simulink model "Antriebsstrangmodell_V1_4_n5"  (R2019a)
settings: Solver=FixedStepAuto  StartTime=0.0  StopTime=t_Simulation  FixedStep=dt  RelTol=1e-3
values from neighbouring files (symbols this model uses):
  A_Stirn = 2    [SIMULA~1.M]    (also in SIMULA~2.M)
  alpha_Luft = -4e-3    (= -0.004)    [SIMULA~1.M]    (also in SIMULA~2.M)
  alpha_Rotor = alpha_Al    (= 0.004)    [SIMULA~1.M]    (also in SIMULA~2.M)
  alpha_Stator = alpha_Al    (= 0.004)    [SIMULA~1.M]    (also in SIMULA~2.M)
  alpha_Ummag = -0.75e-3    (= -0.00075)    [SIMULA~1.M]    (also in SIMULA~2.M)
  c_W = 0.37    [SIMULA~1.M]    (also in SIMULA~2.M)
  COG_x = 1.4267    [SIMULA~1.M]    (also in SIMULA~2.M)
  COG_z = 0.4572    [SIMULA~1.M]    (also in SIMULA~2.M)
  cp_Luft = 1008.8    [SIMULA~1.M]    (also in SIMULA~2.M)
  e_Fahrzeug = 1.0478    [SIMULA~1.M]    (also in SIMULA~2.M)
  eta_EMaschine_Break_M_EMaschine = flipud(KennfeldMaschine.M(:,1))'    [SIMULA~1.M]    (also in SIMULA~2.M)
  eta_EMaschine_Break_M_EMaschine_reku = -KennfeldMaschine.M(:,1)'    [SIMULA~1.M]    (also in SIMULA~2.M)
  eta_EMaschine_Break_n_EMaschine = KennfeldMaschine.n(end-1,:)    [SIMULA~1.M]    (also in SIMULA~2.M)
  eta_EMaschine_Break_n_EMaschine_reku = KennfeldMaschine.n(end-1,:)    [SIMULA~1.M]    (also in SIMULA~2.M)
  eta_EMaschine_Faktor_Volllast = 0.98    [SIMULA~1.M]    (also in SIMULA~2.M)
  eta_EMaschine_Table = flip(KennfeldMaschine.etages,1)    [SIMULA~1.M]    (also in SIMULA~2.M)
  eta_EMaschine_Table_reku = KennfeldMaschine.etages    [SIMULA~1.M]    (also in SIMULA~2.M)
  eta_Getriebe = 0.96    [SIMULA~1.M]    (also in SIMULA~2.M)
  eta_IA = 0.5    [SIMULA~1.M]    (also in SIMULA~2.M)
  h_WC_pumpoff = Nu_WC*lam_WC/dh_WC    [SIMULA~1.M]    (also in SIMULA~2.M)
  h_WC_pumpon = Nu_WC*lam_WC/dh_WC    [SIMULA~1.M]    (also in SIMULA~2.M)
  i_Getriebe = 5.697    [SIMULA~1.M]    (also in SIMULA~2.M)
  krb_Korrektur = 0.53/10    (= 0.053)    [SIMULA~1.M]    (also in SIMULA~2.M)
  lam_Luft = 0.028592    [SIMULA~1.M]    (also in SIMULA~2.M)
  M_EMaschine_max = zeros(2,numel(eta_EMaschine_Break_n_EMaschine))    [SIMULA~1.M]    (also in SIMULA~2.M)
  m_Fahrzeug = 825    [SIMULA~1.M]    (also in SIMULA~2.M)
  m_Zuladung = 80    [SIMULA~1.M]    (also in SIMULA~2.M)
  nue_Luft = 19.230034390524e-6    (= 1.92300343905e-05)    [SIMULA~1.M]    (also in SIMULA~2.M)
  pump_start_limit = 273.15 + 33    (= 306.15)    [SIMULA~1.M]    (also in SIMULA~2.M)
  r_dynamisch = 0.2774    [SIMULA~1.M]    (also in SIMULA~2.M)
  rho_Luft = 1.2    [SIMULA~1.M]    (also in SIMULA~2.M)
  rho_Luft_EM = 1.0468    [SIMULA~1.M]    (also in SIMULA~2.M)
  share_EMaschine_Ummagnet_reku_Table = ser.gen.share_Ummagnetisierungsverluste    [SIMULA~1.M]    (also in SIMULA~2.M)
  share_EMaschine_Ummagnet_Table = ser.mot.share_Ummagnetisierungsverluste    [SIMULA~1.M]    (also in SIMULA~2.M)
  share_EMaschine_Wicklung_reku_Table = ser.gen.share_Wicklungsverluste    [SIMULA~1.M]    (also in SIMULA~2.M)
  share_EMaschine_Wicklung_Table = ser.mot.share_Wicklungsverluste    [SIMULA~1.M]    (also in SIMULA~2.M)
  share_EMaschine_WirkMech_reku_Table = ser.gen.share_WirkmechVerluste    [SIMULA~1.M]    (also in SIMULA~2.M)
  share_EMaschine_WirkMech_Table = ser.mot.share_WirkmechVerluste    [SIMULA~1.M]    (also in SIMULA~2.M)
  share_EMaschine_WirkZus_reku_Table = ser.gen.share_WirkZusVerl    [SIMULA~1.M]    (also in SIMULA~2.M)
  share_EMaschine_WirkZus_Table = ser.mot.share_WirkZusVerl    [SIMULA~1.M]    (also in SIMULA~2.M)
  T_Entwurf_Rotor = 273.15+20    (= 293.15)    [SIMULA~1.M]    (also in SIMULA~2.M)
  T_Entwurf_Stator = 273.15+20    (= 293.15)    [SIMULA~1.M]    (also in SIMULA~2.M)
  t_Simulation = v_Fahrzeug.Time(end)+1    [SIMULA~1.M]    (also in SIMULA~2.M = v_Fahrzeug.Time(end))
  T_Start_EMaschine = 273.15 + 23    (= 296.15)    [SIMULA~1.M]    (also in SIMULA~2.M)
  v_max = 110    [SIMULA~1.M]    (also in SIMULA~2.M)
  WB = 2.96    [SIMULA~1.M]    (also in SIMULA~2.M)
undefined symbols (not defined in the file or in its folder): A_AGP, A_IA, Anteil_Rotor_Ringe, Anteil_Stator, chi_Lager, D_2a, D_2r, delta, f_R, m_RTO, m_RYO, m_SSL_L, m_STO, m_SYO, m_WH_L, n_dis
libraries: fl_lib x440, nesl_utility x106, SimscapeCustomBlocks_lib x45, simulink x3
(part 1 of 5)
settings Model: Creator=Ludwig Stolle  LastModifiedBy=Ludwig Stolle
settings DataIOCC: SaveOutput=off  SignalLogging=off  DSMLogging=off  SaveTime=off  ReturnWorkspaceOutputs=off
settings DebuggingCC: UnconnectedInputMsg=none  UnconnectedOutputMsg=none

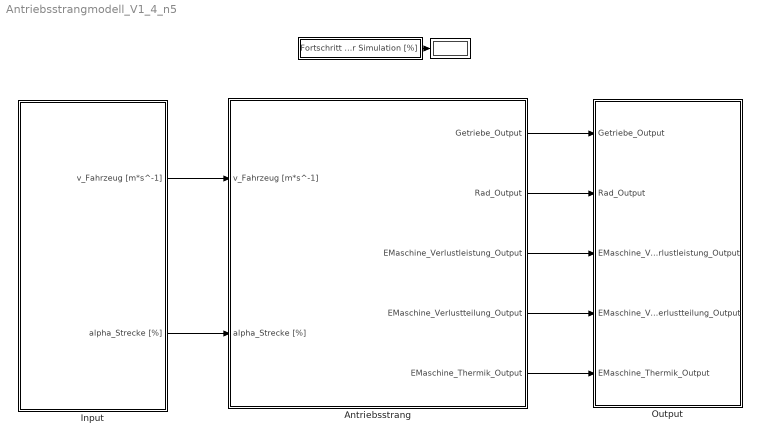
== system Antriebsstrangmodell_V1_4_n5 ==
  "\t\t     " : Subsystem
  " " : Display
      settings: Format=bank
  Antriebsstrang : Subsystem
  Input : Subsystem
  Output : Subsystem
  wires:
  Input/1(v_Fahrzeug [m*s^-1]) -> Antriebsstrang/1(v_Fahrzeug [m*s^-1])
  Input/2(alpha_Strecke [%]) -> Antriebsstrang/2(alpha_Strecke [%])
  Antriebsstrang/1(Getriebe_Output) -> Output/1(Getriebe_Output)
  Antriebsstrang/2(Rad_Output) -> Output/2(Rad_Output)
  "\t\t     "/1(Fortschritt der Simulation [%]) -> " "/1
  Antriebsstrang/3(EMaschine_Verlustleistung_Output) -> Output/3(EMaschine_Verlustleistung_Output)
  Antriebsstrang/4(EMaschine_Verlustteilung_Output) -> Output/4(EMaschine_Verlustteilung_Output)
  Antriebsstrang/5(EMaschine_Thermik_Output) -> Output/5(EMaschine_Thermik_Output)

== system Antriebsstrangmodell_V1_4_n5/		      ==
  note: Fortschritt der Simulation = 100 * simulierte Zeit / t_Simulation
      |
      | mit Fortschritt der Simulation in %
  Clock : Clock
  Constant : Constant  Value=t_Simulation  VectorParams1D=off
  Divide : Product  Inputs=*/
  Umrechnung in % : Gain  Gain=100
  Fortschritt der Simulation [%] : Outport
  wires:
  Constant/1 -> Divide/2
  Clock/1 -> Divide/1
  Divide/1 -> Umrechnung in %/1
  Umrechnung in %/1 -> Fortschritt der Simulation [%]/1

== system Antriebsstrangmodell_V1_4_n5/Antriebsstrang ==
  v_Fahrzeug [m*s^-1] : Inport
  alpha_Strecke [%] : Inport  Port=2
  E-Maschine Thermik : Subsystem
  E-Maschine Verlustleistung : Subsystem
  E-Maschine Verlustteilung : Subsystem
  Getriebe : Subsystem
  Rad : Subsystem
  Getriebe_Output : Outport
  Rad_Output : Outport  Port=2
  EMaschine_Verlustleistung_Output : Outport  Port=3
  EMaschine_Verlustteilung_Output : Outport  Port=4
  EMaschine_Thermik_Output : Outport  Port=5
  wires:
  alpha_Strecke [%]/1 -> Rad/2(alpha_Strecke [%])
  v_Fahrzeug [m*s^-1]/1 -> Rad/1(v_Fahrzeug [m*s^-1])
  Rad/1(Rad_Output) -> Rad_Output/1, Getriebe/1(Rad_Output)
  Getriebe/1(Getriebe_Output) -> Getriebe_Output/1, E-Maschine Verlustleistung/1(Getriebe_Output), E-Maschine Verlustteilung/2(Getriebe_Output), E-Maschine Thermik/2(Getriebe_Output)
  E-Maschine Verlustleistung/1(EMaschine_Verlustleistung_Output) -> EMaschine_Verlustleistung_Output/1, E-Maschine Verlustteilung/1(EMaschine_Verlustleistung_Output)
  E-Maschine Verlustteilung/1(EMaschine_Verlustteilung_Output) -> EMaschine_Verlustteilung_Output/1, E-Maschine Thermik/1(EMaschine_Verlustlteilung_Output)
  E-Maschine Thermik/1(EMaschine_Thermik_Output) -> EMaschine_Thermik_Output/1
  E-Maschine Verlustleistung/2(Regelabweichung [Nm]) -> Rad/3(Regelabweichung [Nm])

== system Antriebsstrangmodell_V1_4_n5/Input ==
  note: Umrechnung km/h in m/s
  note: Nur positive Geschwindigkeit
  From Workspace : FromWorkspace  VariableName=v_Fahrzeug  SampleTime=0  OutputAfterFinalValue=Setting to zero
  From Workspace1 : FromWorkspace  VariableName=alpha_Strecke  SampleTime=0  OutputAfterFinalValue=Setting to zero
  Gain : Gain  Gain=1/3.6
  Saturation : Saturate  UpperLimit=v_max  LowerLimit=0
  v_Fahrzeug [m*s^-1] : Outport
  alpha_Strecke [%] : Outport  Port=2
  wires:
  Saturation/1 -> Gain/1
  From Workspace/1 -> Saturation/1
  Gain/1 -> v_Fahrzeug [m*s^-1]/1
  From Workspace1/1 -> alpha_Strecke [%]/1

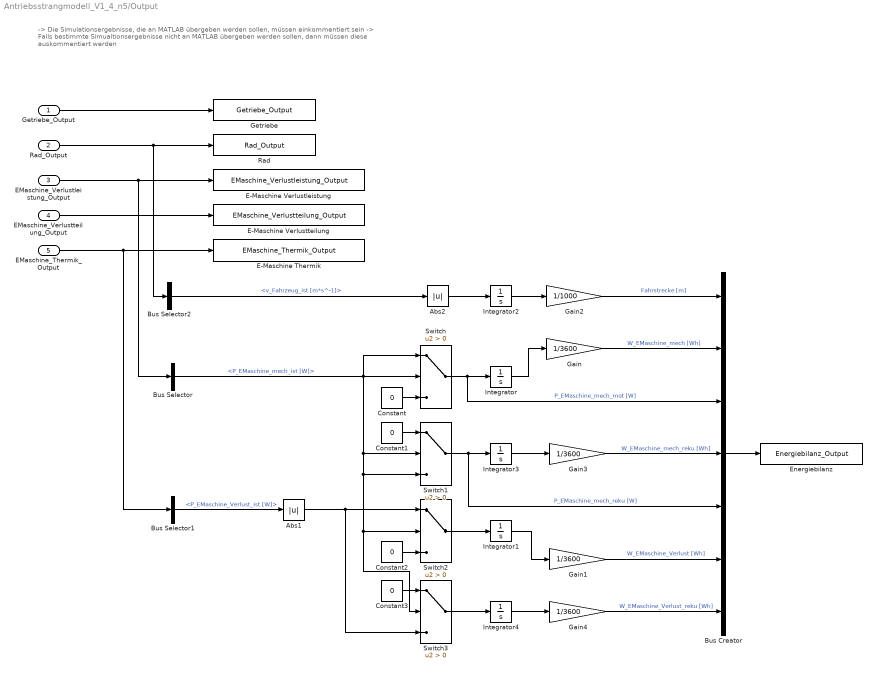
== system Antriebsstrangmodell_V1_4_n5/Output ==
  note: -> Die Simulationsergebnisse, die an MATLAB übergeben werden sollen, müssen einkommentiert sein
      | -> Falls bestimmte Simualtionsergebnisse nicht an MATLAB übergeben werden sollen, dann müssen diese auskommentiert werden
  Getriebe_Output : Inport
  Rad_Output : Inport  Port=2
  EMaschine_Verlustleistung_Output : Inport  Port=3
  EMaschine_Verlustteilung_Output : Inport  Port=4
  EMaschine_Thermik_Output : Inport  Port=5
  Abs1 : Abs
  Abs2 : Abs
  Bus Creator : BusCreator  Inputs=7
  Bus Selector : BusSelector  OutputSignals=P_EMaschine_mech_ist [W]
  Bus Selector1 : BusSelector  OutputSignals=P_EMaschine_Verlust_ist [W]
  Bus Selector2 : BusSelector  OutputSignals=v_Fahrzeug_ist [m*s^-1]
  Constant{,1..3} (4 alike) : Constant  Value=0
  E-Maschine Thermik : ToWorkspace  VariableName=EMaschine_Thermik_Output  SaveFormat=Timeseries  SampleTime=-1
      settings: Decimation=Decimation_Output
  E-Maschine Verlustleistung : ToWorkspace  VariableName=EMaschine_Verlustleistung_Output  SaveFormat=Timeseries  SampleTime=-1
      settings: Decimation=Decimation_Output
  E-Maschine Verlustteilung : ToWorkspace  VariableName=EMaschine_Verlustteilung_Output  SaveFormat=Timeseries  SampleTime=-1
      settings: Decimation=Decimation_Output
  Energiebilanz : ToWorkspace  VariableName=Energiebilanz_Output  SaveFormat=Timeseries  SampleTime=-1
      settings: Decimation=Decimation_Output
  Gain{,1,3..4} (4 alike) : Gain  Gain=1/3600
  Gain2 : Gain  Gain=1/1000
  Getriebe : ToWorkspace  VariableName=Getriebe_Output  SaveFormat=Timeseries  SampleTime=-1
      settings: Decimation=Decimation_Output
  Integrator{,1..4} (5 alike) : Integrator
  Rad : ToWorkspace  VariableName=Rad_Output  SaveFormat=Timeseries  SampleTime=-1
      settings: Decimation=Decimation_Output
  Switch{,1..3} (4 alike) : Switch  Criteria=u2 > Threshold
  wires:
  Getriebe_Output/1 -> Getriebe/1
  Rad_Output/1 -> Rad/1, Bus Selector2/1
  EMaschine_Verlustleistung_Output/1 -> E-Maschine Verlustleistung/1, Bus Selector/1
  EMaschine_Verlustteilung_Output/1 -> E-Maschine Verlustteilung/1
  EMaschine_Thermik_Output/1 -> E-Maschine Thermik/1, Bus Selector1/1
  Bus Selector1/1 -> Abs1/1  "<P_EMaschine_Verlust_ist [W]>"
  Integrator/1 -> Gain/1
  Integrator1/1 -> Gain1/1
  Bus Selector/1 -> Switch/2, Switch3/2, Switch2/2, Switch1/3, Switch1/2, Switch/1  "<P_EMaschine_mech_ist [W]>"
  Bus Creator/1 -> Energiebilanz/1
  Gain/1 -> Bus Creator/2  "W_EMaschine_mech [Wh]"
  Gain2/1 -> Bus Creator/1  "Fahrstrecke [m]"
  Bus Selector2/1 -> Abs2/1  "<v_Fahrzeug_ist [m*s^-1]>"
  Integrator2/1 -> Gain2/1
  Abs2/1 -> Integrator2/1
  Switch/1 -> Bus Creator/3, Integrator/1  "P_EMaschine_mech_mot [W]"
  Constant/1 -> Switch/3
  Constant1/1 -> Switch1/1
  Switch1/1 -> Bus Creator/5, Integrator3/1  "P_EMaschine_mech_reku [W]"
  Integrator3/1 -> Gain3/1
  Gain3/1 -> Bus Creator/4  "W_EMaschine_mech_reku [Wh]"
  Abs1/1 -> Switch3/3, Switch2/1
  Switch2/1 -> Integrator1/1
  Constant2/1 -> Switch2/3
  Gain1/1 -> Bus Creator/6  "W_EMaschine_Verlust [Wh]"
  Constant3/1 -> Switch3/1
  Integrator4/1 -> Gain4/1
  Switch3/1 -> Integrator4/1
  Gain4/1 -> Bus Creator/7  "W_EMaschine_Verlust_reku [Wh]"

== system Antriebsstrangmodell_V1_4_n5/Antriebsstrang/E-Maschine Thermik ==
  EMaschine_Verlustlteilung_Output : Inport
  Getriebe_Output : Inport  Port=2
  Aufteilung mechanischer Verluste auf Lager & Lüftung : Subsystem
  Bus Creator : BusCreator  Inputs=15
  Bus Selector1 : BusSelector  OutputSignals=P_EMaschine_Verlust_Wicklung [W],P_EMaschine_Verlust_Ummagnet [W],P_EMaschine_Verlust_WirkZus [W],P_EMaschine_Verlust_WirkMech [W]
  Bus Selector2 : BusSelector  OutputSignals=n_EMaschine [min^-1]
  Thermisches Netzwerk : Subsystem
  Wärmeübergangskoeffizienten Konvektion Luftspalt und Endcap-Luft : Subsystem
  EMaschine_Thermik_Output : Outport
  wires:
  EMaschine_Verlustlteilung_Output/1 -> Bus Selector1/1
  Getriebe_Output/1 -> Bus Selector2/1
  Bus Creator/1 -> EMaschine_Thermik_Output/1
  Bus Selector2/1 -> Wärmeübergangskoeffizienten Konvektion Luftspalt und Endcap-Luft/1(<n_EMaschine [min^-1]>), Aufteilung mechanischer Verluste auf Lager & Lüftung/2(n_EMaschine [min^-1])  "<n_EMaschine [min^-1]>"
  Bus Selector1/2 -> Thermisches Netzwerk/2(P_EMaschine_Verlust_Ummagnet [W])  "<P_EMaschine_Verlust_Ummagnet [W]>"
  Bus Selector1/3 -> Thermisches Netzwerk/3(P_EMaschine_Verlust_WirkZus [W])  "<P_EMaschine_Verlust_WirkZus [W]>"
  Bus Selector1/1 -> Thermisches Netzwerk/1(P_EMaschine_Verlust_Wicklung [W])  "<P_EMaschine_Verlust_Wicklung [W]>"
  Wärmeübergangskoeffizienten Konvektion Luftspalt und Endcap-Luft/1(HTC_Luftspalt [W*m^-2*K^-1]) -> Thermisches Netzwerk/6(HTC_Luftspalt [W*m^-2*K^-1])
  Aufteilung mechanischer Verluste auf Lager & Lüftung/1(P_EMaschine_Verlust_Lueftung [W]) -> Thermisches Netzwerk/4(P_EMaschine_Verlust_Lueftung [W])
  Bus Selector1/4 -> Aufteilung mechanischer Verluste auf Lager & Lüftung/1(P_EMaschine_Verlust_WirkMech [W])  "<P_EMaschine_Verlust_WirkMech [W]>"
  Aufteilung mechanischer Verluste auf Lager & Lüftung/2(P_EMaschine_Verlust_Lager [W]) -> Thermisches Netzwerk/5(P_EMaschine_Verlust_Lager [W])
  Thermisches Netzwerk/1(T_EMaschine_WH [K]) -> Bus Creator/1
  Thermisches Netzwerk/2(T_EMaschine_Kuehlmittel [K]) -> Bus Creator/2
  Thermisches Netzwerk/3(T_EMaschine_SSL [K]) -> Bus Creator/3
  Thermisches Netzwerk/4(T_EMaschine_ER [K]) -> Bus Creator/4
  Thermisches Netzwerk/5(P_EMaschine_Verlust_ist [W]) -> Bus Creator/5
  Thermisches Netzwerk/6(T_EMaschine_STO [K]) -> Bus Creator/6
  Thermisches Netzwerk/7(T_EMaschine_AGP [K]) -> Bus Creator/7
  Thermisches Netzwerk/8(T_EMaschine_SYO [K]) -> Bus Creator/8
  Thermisches Netzwerk/9(T_EMaschine_RSL [K]) -> Bus Creator/9
  Thermisches Netzwerk/11(T_EMaschine_RYO [K]) -> Bus Creator/11
  Thermisches Netzwerk/10(T_EMaschine_RTO [K]) -> Bus Creator/10
  Wärmeübergangskoeffizienten Konvektion Luftspalt und Endcap-Luft/2(HTC_fconv_Luftspalt [W*m^-2*K^-1]) -> Thermisches Netzwerk/7(HTC_fconv_Luftspalt [W*m^-2*K^-1])
  Wärmeübergangskoeffizienten Konvektion Luftspalt und Endcap-Luft/4(HTC_fconv_Innenluft [W*m^-2*K^-1]) -> Thermisches Netzwerk/9(HTC_fconv_Innenluft [W*m^-2*K^-1])
  Thermisches Netzwerk/12(T_EMaschine_IA [K]) -> Bus Creator/12
  Thermisches Netzwerk/13(T_EMaschine_SH [K]) -> Bus Creator/13
  Thermisches Netzwerk/14(T_EMaschine_HO [K]) -> Bus Creator/14
  Thermisches Netzwerk/15(T_EMaschine_EC [K]) -> Bus Creator/15
  Wärmeübergangskoeffizienten Konvektion Luftspalt und Endcap-Luft/3(HTC_Innenluft [W*m^-2*K^-1]) -> Thermisches Netzwerk/8(HTC_Innenluft [W*m^-2*K^-1])

== system Antriebsstrangmodell_V1_4_n5/Antriebsstrang/E-Maschine Verlustleistung ==
  Getriebe_Output : Inport
  Bus Creator : BusCreator  Inputs=6
  Bus Creator1 : BusCreator  Inputs=6
  Bus Selector : BusSelector  OutputSignals=P_EMaschine_Verlust_korr [W]
  Bus Selector1 : BusSelector  OutputSignals=M_EMaschine [Nm],n_EMaschine [min^-1]
  Compare To Zero : simulink/Logic and Bit Operations/Compare To Zero  relop=>=  OutDataTypeStr=boolean
  Scope : Scope  Commented=on  NumInputPorts=3
  Switch : Switch  Criteria=u2 ~= 0
  Wikrungsgrad und Verlustleistung - Antrieb : Subsystem
  Wikrungsgrad und Verlustleistung - Rekuperation : Subsystem
  EMaschine_Verlustleistung_Output : Outport
  Regelabweichung [Nm] : Outport  Port=2
  wires:
  Getriebe_Output/1 -> Bus Selector1/1
  Bus Selector1/1 -> Wikrungsgrad und Verlustleistung - Antrieb/1(M_EMaschine [Nm]), Compare To Zero/1, Wikrungsgrad und Verlustleistung - Rekuperation/1(M_EMaschine [Nm])  "<M_EMaschine [Nm]>"
  Bus Selector1/2 -> Wikrungsgrad und Verlustleistung - Antrieb/2(n_EMaschine [min^-1]), Wikrungsgrad und Verlustleistung - Rekuperation/2(n_EMaschine [min^-1])  "<n_EMaschine [min^-1]>"
  Wikrungsgrad und Verlustleistung - Antrieb/1(eta_EMaschine [%]) -> Bus Creator/1
  Wikrungsgrad und Verlustleistung - Antrieb/2(P_Leistungselektronik [W]) -> Bus Creator/2
  Wikrungsgrad und Verlustleistung - Antrieb/3(P_EMaschine_Verlust_korr [W]) -> Scope/2, Bus Creator/3
  Wikrungsgrad und Verlustleistung - Rekuperation/1(eta_EMaschine [%]) -> Bus Creator1/1
  Wikrungsgrad und Verlustleistung - Rekuperation/2(P_Leistungselektronik [W]) -> Bus Creator1/2
  Wikrungsgrad und Verlustleistung - Rekuperation/3(P_EMaschine_Verlust_korr [W]) -> Scope/3, Bus Creator1/3
  Bus Creator/1 -> Switch/1
  Bus Creator1/1 -> Switch/3
  Compare To Zero/1 -> Switch/2
  Switch/1 -> Bus Selector/1, EMaschine_Verlustleistung_Output/1
  Bus Selector/1 -> Scope/1  "<P_EMaschine_Verlust_korr [W]>"
  Wikrungsgrad und Verlustleistung - Antrieb/4(P_EMaschine_mech_ist [W]) -> Bus Creator/4
  Wikrungsgrad und Verlustleistung - Rekuperation/4(P_EMaschine_mech_ist [W]) -> Bus Creator1/4
  Wikrungsgrad und Verlustleistung - Antrieb/6(Regelabweichung [Nm]) -> Regelabweichung [Nm]/1, Bus Creator/6, Bus Creator1/6
  Wikrungsgrad und Verlustleistung - Antrieb/5(M_EMaschine_ist [Nm]) -> Bus Creator/5
  Wikrungsgrad und Verlustleistung - Rekuperation/5(M_EMaschine_ist [Nm]) -> Bus Creator1/5

== system Antriebsstrangmodell_V1_4_n5/Antriebsstrang/E-Maschine Verlustteilung ==
  EMaschine_Verlustleistung_Output : Inport
  Getriebe_Output : Inport  Port=2
  Bus Creator : BusCreator  Inputs=4
  Bus Creator1 : BusCreator  Inputs=4
  Bus Selector1 : BusSelector  OutputSignals=P_EMaschine_Verlust_korr [W]
  Bus Selector2 : BusSelector  OutputSignals=M_EMaschine [Nm],n_EMaschine [min^-1]
  Bus Selector3 : BusSelector  Commented=on  OutputSignals=P_Verlust_EMaschine_Wicklung [W],P_Verlust_EMaschine_WirkMech [W]
  Bus Selector4 : BusSelector  Commented=on  OutputSignals=P_Verlust_EMaschine_Wicklung [W],P_Verlust_EMaschine_WirkMech [W]
  Compare To Zero : simulink/Logic and Bit Operations/Compare To Zero  relop=>=  OutDataTypeStr=boolean
  Demux : Demux  Commented=on
  Scope : Scope  Commented=on  NumInputPorts=5
  Scope1 : Scope  Commented=on  NumInputPorts=4
  Switch : Switch  Criteria=u2 ~= 0
  Verlustteilung EMaschine - Antrieb : Subsystem
  Verlustteilung EMaschine - Rekuperation : Subsystem
  EMaschine_Verlustteilung_Output : Outport
  wires:
  EMaschine_Verlustleistung_Output/1 -> Bus Selector1/1
  Getriebe_Output/1 -> Bus Selector2/1
  Bus Selector1/1 -> Verlustteilung EMaschine - Rekuperation/1(<P_Verlust_EMaschine [W]>), Verlustteilung EMaschine - Antrieb/1(<P_Verlust_EMaschine_korr [W]>)  "<P_EMaschine_Verlust_korr [W]>"
  Bus Selector2/1 -> Verlustteilung EMaschine - Rekuperation/2(<M_EMaschine [Nm]>), Compare To Zero/1, Verlustteilung EMaschine - Antrieb/2(<M_EMaschine [Nm]>)  "<M_EMaschine [Nm]>"
  Bus Selector2/2 -> Verlustteilung EMaschine - Antrieb/3(<n_EMaschine [min^-1]>), Verlustteilung EMaschine - Rekuperation/3(<n_EMaschine [min^-1]>)  "<n_EMaschine [min^-1]>"
  Verlustteilung EMaschine - Antrieb/1(P_EMaschine_Verlust_Wicklung [W]) -> Bus Creator/1
  Verlustteilung EMaschine - Antrieb/2(P_EMaschine_Verlust_Ummagnet [W]) -> Bus Creator/2
  Verlustteilung EMaschine - Antrieb/3(P_EMaschine_Verlust_WirkZus [W]) -> Bus Creator/3
  Compare To Zero/1 -> Switch/2
  Switch/1 -> EMaschine_Verlustteilung_Output/1
  Bus Creator/1 -> Switch/1
  Verlustteilung EMaschine - Rekuperation/1(P_EMaschine_Verlust_Wicklung [W]) -> Bus Creator1/1
  Verlustteilung EMaschine - Rekuperation/2(P_EMaschine_Verlust_Ummagnet [W]) -> Bus Creator1/2
  Verlustteilung EMaschine - Rekuperation/3(P_EMaschine_Verlust_WirkZus [W]) -> Bus Creator1/3
  Bus Creator1/1 -> Switch/3
  Demux/4 -> Scope/5
  Demux/1 -> Scope/2
  Demux/2 -> Scope/3
  Demux/3 -> Scope/4
  Bus Selector3/1 -> Scope1/1  "<P_Verlust_EMaschine_Wicklung [W]>"
  Bus Selector4/1 -> Scope1/2  "<P_Verlust_EMaschine_Wicklung [W]>"
  Bus Selector3/2 -> Scope1/3  "<P_Verlust_EMaschine_WirkMech [W]>"
  Bus Selector4/2 -> Scope1/4  "<P_Verlust_EMaschine_WirkMech [W]>"
  Verlustteilung EMaschine - Rekuperation/4(P_EMaschine_Verlust_WirkMech [W]) -> Bus Creator1/4  "P_EMaschine_Verlust_WirkMech [W]"
  Verlustteilung EMaschine - Antrieb/4(P_EMaschine_Verlust_WirkMech [W]) -> Bus Creator/4  "P_EMaschine_Verlust_WirkMech [W]"

== system Antriebsstrangmodell_V1_4_n5/Antriebsstrang/Getriebe ==
  note: Schalter für S1-Betrieb umlegen!
  note: Momentenvorgabe für S1-Kennfeld Berechnung.
  Rad_Output : Inport
  Antreiben : Subsystem
  Bus Creator : BusCreator  Inputs=4
  Bus Creator1 : BusCreator  Inputs=4
  Bus Creator2 : BusCreator  Inputs=4
  Bus Selector : BusSelector  OutputSignals=n_Rad [min^-1],M_Rad [Nm],P_Rad [W]
  Bus Selector1 : BusSelector  OutputSignals=n_EMaschine [min^-1],P_EMaschine [W],P_Verlust_Getriebe [W],M_EMaschine [Nm]
  Compare To Zero : simulink/Logic and Bit Operations/Compare To Zero  relop=>=  OutDataTypeStr=boolean
  From Workspace1 : FromWorkspace  VariableName=M_EM  SampleTime=0  OutputAfterFinalValue=Setting to zero
  Manual Switch : ManualSwitch
  Rekuperieren : Subsystem
  Switch : Switch  Criteria=u2 ~= 0
  Getriebe_Output : Outport
  wires:
  Rad_Output/1 -> Bus Selector/1
  Bus Selector/1 -> Rekuperieren/1(n_Rad [min^-1]), Antreiben/1(n_Rad [min^-1])  "<n_Rad [min^-1]>"
  Bus Selector/2 -> Compare To Zero/1, Rekuperieren/2(M_Rad [Nm]), Antreiben/2(M_Rad [Nm])  "<M_Rad [Nm]>"
  Bus Selector/3 -> Rekuperieren/3(P_Rad [W]), Antreiben/3(P_Rad [W])  "<P_Rad [W]>"
  Antreiben/1(n_EMaschine [min^-1]) -> Bus Creator/1
  Antreiben/2(M_EMaschine [Nm]) -> Bus Creator/2
  Antreiben/3(P_EMaschine [W]) -> Bus Creator/3
  Antreiben/4(P_Verlust_Getriebe [W]) -> Bus Creator/4
  Rekuperieren/3(P_EMaschine [W]) -> Bus Creator1/3
  Rekuperieren/1(n_EMaschine [min^-1]) -> Bus Creator1/1
  Rekuperieren/4(P_Verlust_Getriebe [W]) -> Bus Creator1/4
  Rekuperieren/2(M_EMaschine [Nm]) -> Bus Creator1/2
  Compare To Zero/1 -> Switch/2
  Bus Creator/1 -> Switch/1
  Bus Creator1/1 -> Switch/3
  Switch/1 -> Bus Selector1/1
  Bus Selector1/4 -> Manual Switch/1  "<M_EMaschine [Nm]>"
  Manual Switch/1 -> Bus Creator2/4  "M_EMaschine [Nm]"
  Bus Selector1/1 -> Bus Creator2/1  "<n_EMaschine [min^-1]>"
  Bus Selector1/2 -> Bus Creator2/2  "<P_EMaschine [W]>"
  Bus Selector1/3 -> Bus Creator2/3  "<P_Verlust_Getriebe [W]>"
  Bus Creator2/1 -> Getriebe_Output/1
  From Workspace1/1 -> Manual Switch/2

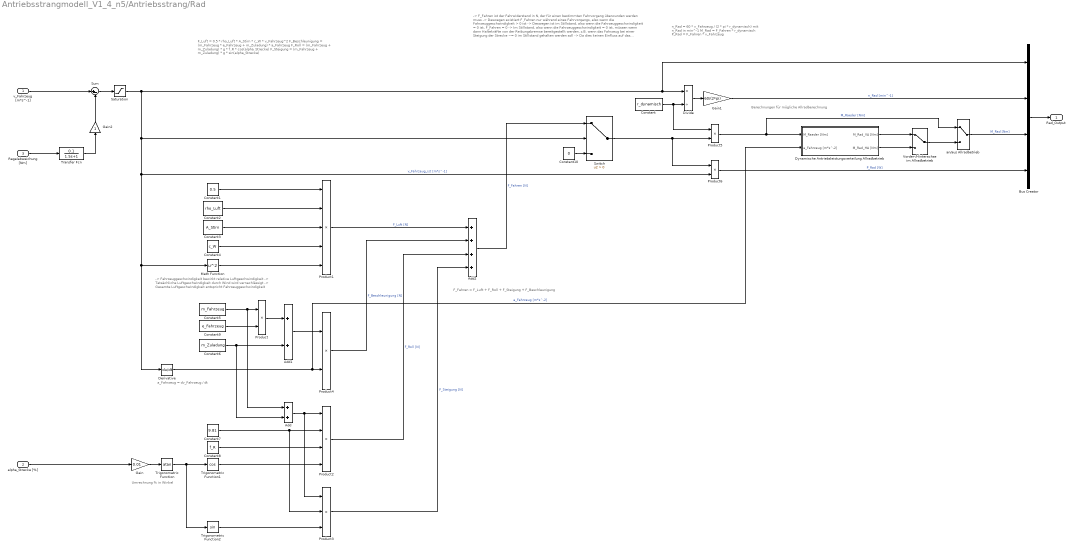
== system Antriebsstrangmodell_V1_4_n5/Antriebsstrang/Rad ==
  note: Berechnungen für mögliche Allradberechnung
  note: -> F_Fahren ist der Fahrwiderstand in N, der für einen bestimmten Fahrvorgang überwunden werden muss
      | -> Deswegen existiert F_Fahren nur während eines Fahrvorgangs, also wenn die Fahrzeuggeschwindigkeit > 0 ist
      | -> Deswegen ist im Stillstand, also wenn die Fahrzeuggeschwindigkeit = 0 ist, F_Fahren = 0
      |
      | -> Im Stillstand, also wenn die Fahrzeuggeschwindigkeit = 0 ist, müssen wenn dann Haltekräfte von der Reibungsbremse bereitgestellt werden, z.B. wenn das Fahrzeug bei einer Steigung der Strecke ~= 0 im Stillstand gehalten werden soll
      | -> Da dies keinen Einfluss auf das Thermomanagementsystem eines Fahrzeugs hat, werden mögliche Haltekräfte im Thermomanagamentsystemmodell nicht betrachtet
      | -> Da das Moment an den Rädern und die Leistungsanforderung an die Räder nur abh. von F_Fahren berechnet werden, werden an den Rädern nur Momente und Leistungsanforderungen aus dem Fahrbetrieb betrachtet, nicht jedoch aus dem Stillstandsbetrieb
  note: n_Rad = 60 * v_Fahrzeug / (2 * pi * r_dynamisch)
      | mit n_Rad in min^-1
      |
      | M_Rad = F_Fahren * r_dynamisch
      |
      | P_Rad = F_Fahren * v_Fahrzeug
  note: F_Luft = 0.5 * rho_Luft * A_Stirn * c_W * v_Fahrzeug^2
      |
      | F_Beschleunigung = (m_Fahrzeug * e_Fahrzeug + m_Zuladung) * a_Fahrzeug
      |
      | F_Roll = (m_Fahrzeug + m_Zuladung) * g * f_R * cos(alpha_Strecke)
      |
      | F_Steigung = (m_Fahrzeug + m_Zuladung) * g * sin(alpha_Strecke)
  note: F_Fahren = F_Luft + F_Roll + F_Steigung + F_Beschleunigung
  note: -> Fahrzeuggeschwindigkeit bewirkt relative Luftgeschwindigkeit
      | -> Tatsächliche Luftgeschwindigkeit durch Wind wird vernachlässigt
      | -> Gesamte Luftgeschwindigkeit entspricht Fahrzeuggeschwindigkeit
  note: a_Fahrzeug = dv_Fahrzeug / dt
  note: Umrechnung % in Winkel
  v_Fahrzeug [m*s^-1] : Inport
  alpha_Strecke [%] : Inport  Port=2
  Regelabweichung [Nm] : Inport  Port=3
  Add : Sum
  Add1 : Sum
  Add2 : Sum  Inputs=4
  Bus Creator : BusCreator  Inputs=4
  Constant : Constant  Value=r_dynamisch  VectorParams1D=off
  Constant1 : Constant  Value=0.5  VectorParams1D=off
  Constant10 : Constant  Value=0  VectorParams1D=off
  Constant2 : Constant  Value=rho_Luft  VectorParams1D=off
  Constant3 : Constant  Value=A_Stirn  VectorParams1D=off
  Constant4 : Constant  Value=c_W  VectorParams1D=off
  Constant5 : Constant  Value=m_Fahrzeug  VectorParams1D=off
  Constant6 : Constant  Value=m_Zuladung  VectorParams1D=off
  Constant7 : Constant  Value=9.81  VectorParams1D=off
  Constant8 : Constant  Value=f_R  VectorParams1D=off
  Constant9 : Constant  Value=e_Fahrzeug  VectorParams1D=off
  Derivative : Derivative
  Divide : Product  Inputs=*/
  Dynamische Antriebsleistungsverteilung Allradbetrieb : Subsystem
  Gain : Gain  Gain=0.01
  Gain1 : Gain  Gain=60/(2*pi)
  Gain2 : Gain
  Math Function : Math  Operator=square  SaturateOnIntegerOverflow=on
  Product{,4..6} (4 alike) : Product
  Product1 : Product  Inputs=5
  Product2 : Product  Inputs=4
  Product3 : Product  Inputs=3
  Saturation : Saturate  UpperLimit=v_max/3.6  LowerLimit=0
  Sum : Sum  Inputs=|+-
  Switch : Switch  Criteria=u2 > Threshold
  Transfer Fcn : TransferFcn  Numerator=[0.1]  Denominator=[1.5 1]
  Trigonometric Function : Trigonometry  Operator=atan
  Trigonometric Function1 : Trigonometry  Operator=cos
  Trigonometric Function2 : Trigonometry
  Vorder-/Hinterachse im Allradbetrieb : ManualSwitch
  an/aus Allradbetrieb : ManualSwitch
  Rad_Output : Outport
  wires:
  Product6/1 -> Bus Creator/4  "P_Rad [W]"
  Constant5/1 -> Add/1, Product/1
  Constant6/1 -> Add1/2, Add/2
  Constant9/1 -> Product/2
  Product/1 -> Add1/1
  Derivative/1 -> Dynamische Antriebsleistungsverteilung Allradbetrieb/2(a_Fahrzeug [m*s^-2]), Product4/2  "a_Fahrzeug [m*s^-2]"
  Add1/1 -> Product4/1
  Product1/1 -> Add2/1  "F_Luft [N]"
  Product4/1 -> Add2/2  "F_Beschleunigung [N]"
  Trigonometric Function/1 -> Trigonometric Function2/1, Trigonometric Function1/1
  Add/1 -> Product3/1, Product2/1
  Constant7/1 -> Product3/2, Product2/2
  Trigonometric Function2/1 -> Product3/3
  Product3/1 -> Add2/4  "F_Steigung [N]"
  Trigonometric Function1/1 -> Product2/4
  Constant8/1 -> Product2/3
  Product2/1 -> Add2/3  "F_Roll [N]"
  alpha_Strecke [%]/1 -> Gain/1
  Gain/1 -> Trigonometric Function/1
  Constant/1 -> Divide/2, Product5/1
  Divide/1 -> Gain1/1
  Gain1/1 -> Bus Creator/2  "n_Rad [min^-1]"
  Bus Creator/1 -> Rad_Output/1
  Constant3/1 -> Product1/3
  Constant1/1 -> Product1/1
  Constant2/1 -> Product1/2
  Constant4/1 -> Product1/4
  Math Function/1 -> Product1/5
  Add2/1 -> Switch/1  "F_Fahren [N]"
  Constant10/1 -> Switch/3
  Switch/1 -> Product5/2, Product6/1
  Saturation/1 -> Bus Creator/1, Divide/1, Product6/2, Math Function/1, Derivative/1, Switch/2  "v_Fahrzeug_ist [m*s^-1]"
  Sum/1 -> Saturation/1
  v_Fahrzeug [m*s^-1]/1 -> Sum/1
  Regelabweichung [Nm]/1 -> Transfer Fcn/1
  Transfer Fcn/1 -> Gain2/1
  Gain2/1 -> Sum/2
  Product5/1 -> an/aus Allradbetrieb/1, Dynamische Antriebsleistungsverteilung Allradbetrieb/1(M_Raeder [Nm])  "M_Raeder [Nm]"
  an/aus Allradbetrieb/1 -> Bus Creator/3  "M_Rad [Nm]"
  Dynamische Antriebsleistungsverteilung Allradbetrieb/2(M_Rad_HA [Nm]) -> Vorder-/Hinterachse im Allradbetrieb/2
  Dynamische Antriebsleistungsverteilung Allradbetrieb/1(M_Rad_VA [Nm]) -> Vorder-/Hinterachse im Allradbetrieb/1
  Vorder-/Hinterachse im Allradbetrieb/1 -> an/aus Allradbetrieb/2

== system Antriebsstrangmodell_V1_4_n5/Antriebsstrang/E-Maschine Thermik/Aufteilung mechanischer Verluste auf Lager & Lüftung ==
  note: Berechnung der Anteile von Luftwiderstand und Lagerverlusten an ges. mechanischem Verlust nach CHIN 2018.
      | Verluste sind nur von der Drehzahl abhängig. Daher normierte Verluste angenähert mittels Polynom 2. Grades für Luftwiderstand
      | und Polynom 1. Grades für Lagerreibung.
  P_EMaschine_Verlust_WirkMech [W] : Inport
  n_EMaschine [min^-1] : Inport  Port=2
  Abs : Abs
  Add1 : Sum  Inputs=+-
  Anteil Lagerverluste an mechanischen Verlusten : Lookup_n-D  NumberOfTableDimensions=1  BreakpointsForDimension1=chi_Lager(1,:)  BeginIndexSearchUsingPreviousIndexResult=on  Table=chi_Lager(2,:)  ExtrapMethod=Clip  UseLastTableValue=on  InternalRulePriority=Speed  RndMeth=Simplest  InputSameDT=on
  Divide1 : Product  Inputs=**
  P_EMaschine_Verlust_Lueftung [W] : Outport
  P_EMaschine_Verlust_Lager [W] : Outport  Port=2
  wires:
  n_EMaschine [min^-1]/1 -> Abs/1
  Abs/1 -> Anteil Lagerverluste an mechanischen Verlusten/1
  P_EMaschine_Verlust_WirkMech [W]/1 -> Divide1/1, Add1/1
  Anteil Lagerverluste an mechanischen Verlusten/1 -> Divide1/2  "Anteil Lagerverluste am gesamten mechanischen Verlust"
  Divide1/1 -> Add1/2, P_EMaschine_Verlust_Lager [W]/1  "P_EMaschine_Verlust_Lager [W]"
  Add1/1 -> P_EMaschine_Verlust_Lueftung [W]/1  "P_EMaschine_Verlust_Lueftung [W]"
